simulink model "mdl_4reac_2pump"  (R2020b)
settings: Solver=FixedStepAuto  StartTime=0.0  StopTime=1000  FixedStep=h  MaxStep=1  RelTol=1e-3  AbsTol=1e-6
undefined symbols (not defined in the file or in its folder): p_4reac_2pump
settings Model: PacingRate=0.100000  Creator=nobel  LastModifiedBy=natha

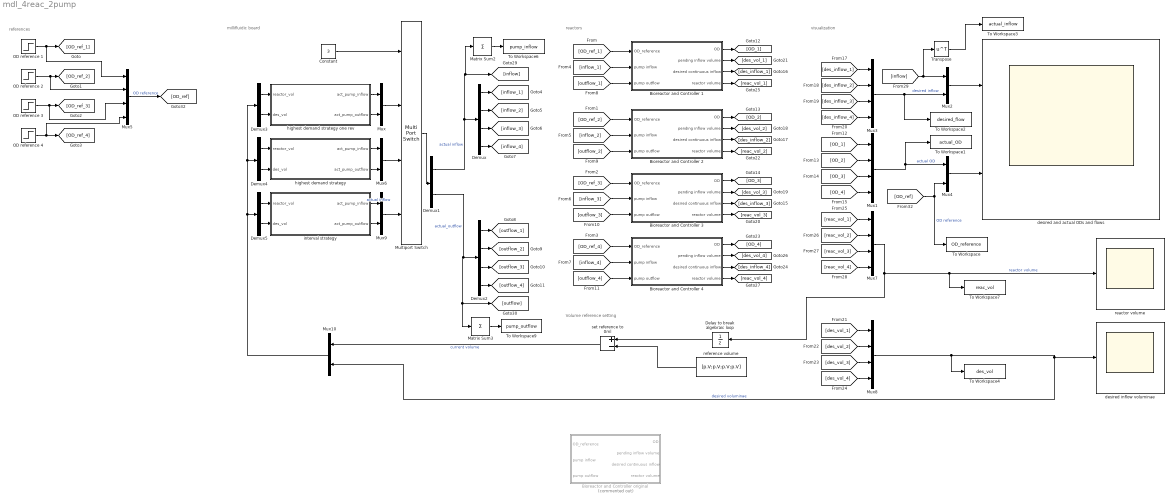
== system mdl_4reac_2pump ==
  note: Volume reference setting
  note: visualization
  note: reactors
  note: millifluidic board
  note: references
  Bioreactor and Controller 1 : Subsystem  mask{p=p_4reac_2pump}
      mask prompts: p "Reactor Parameter Struct"
  Bioreactor and Controller 2 : Subsystem  mask{p=p_4reac_2pump}
      mask prompts: p "Reactor Parameter Struct"
  Bioreactor and Controller 3 : Subsystem  mask{p=p_4reac_2pump}
      mask prompts: p "Reactor Parameter Struct"
  Bioreactor and Controller 4 : Subsystem  mask{p=p_4reac_2pump}
      mask prompts: p "Reactor Parameter Struct"
  Bioreactor and Controller original : Subsystem  Commented=on  mask{p=p_4reac_2pump}
      mask prompts: p "Reactor Parameter Struct"
  Constant : Constant  Value=3
  Delay to break algebraic loop : UnitDelay  InitialCondition=[15; 15; 15; 15]  SampleTime=-1  HasFrameUpgradeWarning=on
  Demux : Demux
  Demux{1,3..5} (4 alike) : Demux  Outputs=2
  Demux2 : Demux
  Matrix Sum2 : Sum  Inputs=+
  Matrix Sum3 : Sum  Inputs=+
  Multiport Switch : MultiPortSwitch
  Mux{,2,4,6,9..10} (6 alike) : Mux  Inputs=2
  Mux{1,3,5,7..8} (5 alike) : Mux
  OD reference 1 : Step  Time=p.r1.step_time  Before=p.r1.init_val  After=p.r1.final_val  SampleTime=0  mask{p=p_4reac_2pump}
      mask prompts: p "Reactor Parameter Struct"
  OD reference 2 : Step  Time=p.r2.step_time  Before=p.r2.init_val  After=p.r2.final_val  SampleTime=0  mask{p=p_4reac_2pump}
      mask prompts: p "Reactor Parameter Struct"
  OD reference 3 : Step  Time=p.r3.step_time  Before=p.r3.init_val  After=p.r3.final_val  SampleTime=0  mask{p=p_4reac_2pump}
      mask prompts: p "Reactor Parameter Struct"
  OD reference 4 : Step  Time=p.r4.step_time  Before=p.r4.init_val  After=p.r4.final_val  SampleTime=0  mask{p=p_4reac_2pump}
      mask prompts: p "Reactor Parameter Struct"
  To Workspace : ToWorkspace  VariableName=OD_reference  SampleTime=-1
  To Workspace1 : ToWorkspace  VariableName=actual_OD  SampleTime=-1
  To Workspace2 : ToWorkspace  VariableName=desired_flow  SampleTime=-1
  To Workspace3 : ToWorkspace  VariableName=actual_inflow  SampleTime=-1
      settings: Save2DSignal=2-D array (concatenate along first dimension)
  To Workspace4 : ToWorkspace  VariableName=des_vol  SampleTime=-1
  To Workspace6 : ToWorkspace  VariableName=pump_inflow  SampleTime=-1
      settings: Save2DSignal=2-D array (concatenate along first dimension)
  To Workspace7 : ToWorkspace  VariableName=reac_vol  SampleTime=-1
  To Workspace9 : ToWorkspace  VariableName=pump_outflow  SampleTime=-1
      settings: Save2DSignal=2-D array (concatenate along first dimension)
  Transpose : Math  Operator=transpose  SaturateOnIntegerOverflow=on
  desired and actual ODs and flows : Scope  NumInputPorts=2
  desired inflow voluminae : Scope
  highest demand strategy : Stateflow chart  TreatAsAtomicUnit=on  mask{p=p_4reac_2pump}
      mask prompts: p "Reactor Parameter Struct"
  highest demand strategy one rev : Stateflow chart  TreatAsAtomicUnit=on  mask{p=p_4reac_2pump}
      mask prompts: p "Reactor Parameter Struct"
  interval strategy : Stateflow chart  TreatAsAtomicUnit=on  mask{p=p_4reac_2pump}
      mask prompts: p "Reactor Parameter Struct"
  reactor volume : Scope
  reference volume : Constant  Value=[p.V;p.V;p.V;p.V]  mask{p=p_4reac_2pump}
      mask prompts: p "Reactor Parameter Struct"
  set reference to 0ml : Sum  Inputs=+-
  wires:
  Bioreactor and Controller 1/2(pending inflow volume) -> [des_vol_1]
  Mux8/1 -> To Workspace4/1, Mux10/2, desired inflow voluminae/1  "desired voluminae"
  Mux1/1 -> To Workspace1/1, Mux4/1  "actual OD"
  Mux2/1 -> desired and actual ODs and flows/1
  Mux3/1 -> To Workspace2/1, Mux2/2  "desired inflow"
  Mux4/1 -> desired and actual ODs and flows/2
  Mux5/1 -> [OD_ref]  "OD reference"
  Demux1/1 -> Matrix Sum2/1, [inflow], Demux/1  "actual inflow"
  Mux7/1 -> Delay to break algebraic loop/1, To Workspace7/1, reactor volume/1  "reactor volume"
  reference volume/1 -> set reference to 0ml/2
  OD reference 1/1 -> Mux5/1, [OD_ref_1]
  OD reference 2/1 -> Mux5/2, [OD_ref_2]
  OD reference 3/1 -> Mux5/3, [OD_ref_3]
  OD reference 4/1 -> Mux5/4, [OD_ref_4]
  [OD_ref_1] -> Bioreactor and Controller 1/1(OD_reference)
  [OD_ref_2] -> Bioreactor and Controller 2/1(OD_reference)
  [OD_ref_3] -> Bioreactor and Controller 3/1(OD_reference)
  [OD_ref_4] -> Bioreactor and Controller 4/1(OD_reference)
  Demux/1 -> [inflow_1]
  Demux/2 -> [inflow_2]
  Demux/3 -> [inflow_3]
  Demux/4 -> [inflow_4]
  [inflow_1] -> Bioreactor and Controller 1/2(pump inflow)
  [inflow_2] -> Bioreactor and Controller 2/2(pump inflow)
  [inflow_3] -> Bioreactor and Controller 3/2(pump inflow)
  [inflow_4] -> Bioreactor and Controller 4/2(pump inflow)
  Demux2/4 -> [outflow_4]
  Demux2/3 -> [outflow_3]
  Demux2/2 -> [outflow_2]
  Demux2/1 -> [outflow_1]
  [outflow_1] -> Bioreactor and Controller 1/3(pump outflow)
  [outflow_2] -> Bioreactor and Controller 2/3(pump outflow)
  [outflow_3] -> Bioreactor and Controller 3/3(pump outflow)
  [outflow_4] -> Bioreactor and Controller 4/3(pump outflow)
  Bioreactor and Controller 1/1(OD) -> [OD_1]
  [OD_1] -> Mux1/1
  [OD_2] -> Mux1/2
  [OD_3] -> Mux1/3
  [OD_4] -> Mux1/4
  [des_inflow_1] -> Mux3/1
  [des_inflow_2] -> Mux3/2
  [des_inflow_3] -> Mux3/3
  [des_inflow_4] -> Mux3/4
  [des_vol_4] -> Mux8/4
  [des_vol_3] -> Mux8/3
  [des_vol_2] -> Mux8/2
  [des_vol_1] -> Mux8/1
  Bioreactor and Controller 1/4(reactor volume) -> [reac_vol_1]
  [reac_vol_1] -> Mux7/1
  [reac_vol_2] -> Mux7/2
  [reac_vol_3] -> Mux7/3
  [reac_vol_4] -> Mux7/4
  Demux1/2 -> Matrix Sum3/1, [outflow], Demux2/1  "actual_outflow"
  [inflow] -> Transpose/1, Mux2/1
  [OD_ref] -> To Workspace/1, Mux4/2  "OD reference"
  Transpose/1 -> To Workspace3/1
  set reference to 0ml/1 -> Mux10/1  "current volume"
  Delay to break algebraic loop/1 -> set reference to 0ml/1
  Bioreactor and Controller 1/3(desired continuous inflow) -> [des_inflow_1]
  Bioreactor and Controller 2/3(desired continuous inflow) -> [des_inflow_2]
  Bioreactor and Controller 2/4(reactor volume) -> [reac_vol_2]
  Bioreactor and Controller 2/1(OD) -> [OD_2]
  Bioreactor and Controller 2/2(pending inflow volume) -> [des_vol_2]
  Bioreactor and Controller 3/2(pending inflow volume) -> [des_vol_3]
  Bioreactor and Controller 3/1(OD) -> [OD_3]
  Bioreactor and Controller 3/4(reactor volume) -> [reac_vol_3]
  Bioreactor and Controller 3/3(desired continuous inflow) -> [des_inflow_3]
  Bioreactor and Controller 4/3(desired continuous inflow) -> [des_inflow_4]
  Bioreactor and Controller 4/4(reactor volume) -> [reac_vol_4]
  Bioreactor and Controller 4/1(OD) -> [OD_4]
  Bioreactor and Controller 4/2(pending inflow volume) -> [des_vol_4]
  Matrix Sum2/1 -> To Workspace6/1
  Matrix Sum3/1 -> To Workspace9/1
  Multiport Switch/1 -> Demux1/1
  highest demand strategy one rev/1(act_pump_inflow) -> Mux/1
  highest demand strategy one rev/2(act_pump_outflow) -> Mux/2
  highest demand strategy/1(act_pump_inflow) -> Mux6/1
  highest demand strategy/2(act_pump_outflow) -> Mux6/2
  interval strategy/1(act_pump_inflow) -> Mux9/1  "actual inflow"
  interval strategy/2(act_pump_outflow) -> Mux9/2
  Mux/1 -> Multiport Switch/2
  Mux6/1 -> Multiport Switch/3
  Mux9/1 -> Multiport Switch/4
  Demux3/1 -> highest demand strategy one rev/1(reactor_vol)
  Demux3/2 -> highest demand strategy one rev/2(des_vol)
  Demux4/1 -> highest demand strategy/1(reactor_vol)
  Demux4/2 -> highest demand strategy/2(des_vol)
  Demux5/1 -> interval strategy/1(reactor_vol)
  Demux5/2 -> interval strategy/2(des_vol)
  Mux10/1 -> Demux5/1, Demux4/1, Demux3/1
  Constant/1 -> Multiport Switch/1

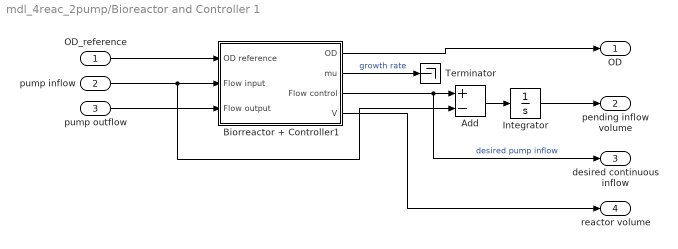
== system mdl_4reac_2pump/Bioreactor and Controller 1 ==
  OD_reference : Inport
  pump inflow : Inport  Port=2
  pump outflow : Inport  Port=3
  Add : Sum  Inputs=+-
  Biorreactor + Controller1 : Subsystem
  Integrator : Integrator
  Terminator : Terminator
  OD : Outport
  pending inflow volume : Outport  Port=2
  desired continuous inflow : Outport  Port=3
  reactor volume : Outport  Port=4
  wires:
  OD_reference/1 -> Biorreactor + Controller1/1(OD reference)
  Biorreactor + Controller1/2(mu) -> Terminator/1  "growth rate"
  Biorreactor + Controller1/1(OD) -> OD/1
  Biorreactor + Controller1/3(Flow control) -> desired continuous inflow/1, Add/1  "desired pump inflow"
  pump inflow/1 -> Add/2, Biorreactor + Controller1/2(Flow input)
  Biorreactor + Controller1/4(V) -> reactor volume/1
  pump outflow/1 -> Biorreactor + Controller1/3(Flow output)
  Add/1 -> Integrator/1
  Integrator/1 -> pending inflow volume/1

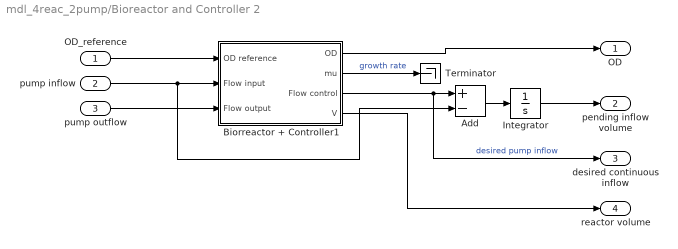
== system mdl_4reac_2pump/Bioreactor and Controller 2 ==
  OD_reference : Inport
  pump inflow : Inport  Port=2
  pump outflow : Inport  Port=3
  Add : Sum  Inputs=+-
  Biorreactor + Controller1 : Subsystem
  Integrator : Integrator
  Terminator : Terminator
  OD : Outport
  pending inflow volume : Outport  Port=2
  desired continuous inflow : Outport  Port=3
  reactor volume : Outport  Port=4
  wires:
  Integrator/1 -> pending inflow volume/1
  Add/1 -> Integrator/1
  pump outflow/1 -> Biorreactor + Controller1/3(Flow output)
  Biorreactor + Controller1/4(V) -> reactor volume/1
  pump inflow/1 -> Biorreactor + Controller1/2(Flow input), Add/2
  Biorreactor + Controller1/3(Flow control) -> Add/1, desired continuous inflow/1  "desired pump inflow"
  Biorreactor + Controller1/1(OD) -> OD/1
  Biorreactor + Controller1/2(mu) -> Terminator/1  "growth rate"
  OD_reference/1 -> Biorreactor + Controller1/1(OD reference)

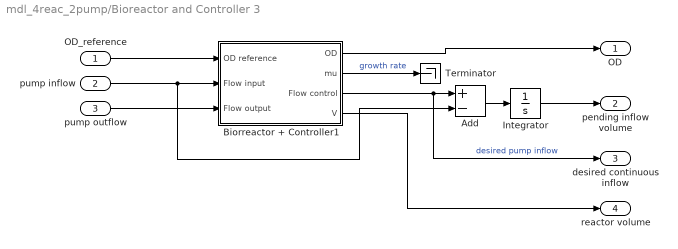
== system mdl_4reac_2pump/Bioreactor and Controller 3 ==
  OD_reference : Inport
  pump inflow : Inport  Port=2
  pump outflow : Inport  Port=3
  Add : Sum  Inputs=+-
  Biorreactor + Controller1 : Subsystem
  Integrator : Integrator
  Terminator : Terminator
  OD : Outport
  pending inflow volume : Outport  Port=2
  desired continuous inflow : Outport  Port=3
  reactor volume : Outport  Port=4
  wires:
  OD_reference/1 -> Biorreactor + Controller1/1(OD reference)
  Biorreactor + Controller1/2(mu) -> Terminator/1  "growth rate"
  Biorreactor + Controller1/1(OD) -> OD/1
  Biorreactor + Controller1/3(Flow control) -> desired continuous inflow/1, Add/1  "desired pump inflow"
  pump inflow/1 -> Add/2, Biorreactor + Controller1/2(Flow input)
  Biorreactor + Controller1/4(V) -> reactor volume/1
  pump outflow/1 -> Biorreactor + Controller1/3(Flow output)
  Add/1 -> Integrator/1
  Integrator/1 -> pending inflow volume/1

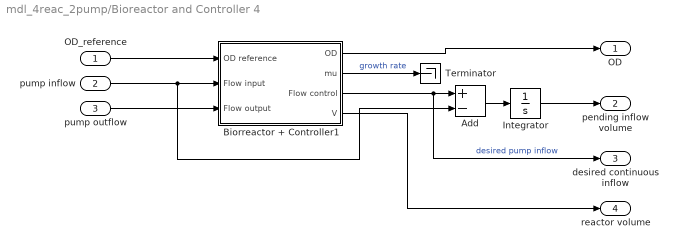
== system mdl_4reac_2pump/Bioreactor and Controller 4 ==
  OD_reference : Inport
  pump inflow : Inport  Port=2
  pump outflow : Inport  Port=3
  Add : Sum  Inputs=+-
  Biorreactor + Controller1 : Subsystem
  Integrator : Integrator
  Terminator : Terminator
  OD : Outport
  pending inflow volume : Outport  Port=2
  desired continuous inflow : Outport  Port=3
  reactor volume : Outport  Port=4
  wires:
  Integrator/1 -> pending inflow volume/1
  Add/1 -> Integrator/1
  pump outflow/1 -> Biorreactor + Controller1/3(Flow output)
  Biorreactor + Controller1/4(V) -> reactor volume/1
  pump inflow/1 -> Biorreactor + Controller1/2(Flow input), Add/2
  Biorreactor + Controller1/3(Flow control) -> Add/1, desired continuous inflow/1  "desired pump inflow"
  Biorreactor + Controller1/1(OD) -> OD/1
  Biorreactor + Controller1/2(mu) -> Terminator/1  "growth rate"
  OD_reference/1 -> Biorreactor + Controller1/1(OD reference)

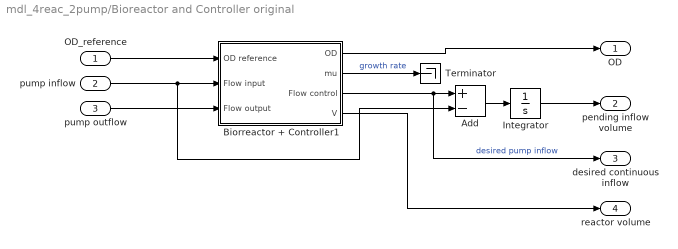
== system mdl_4reac_2pump/Bioreactor and Controller original ==
  OD_reference : Inport
  pump inflow : Inport  Port=2
  pump outflow : Inport  Port=3
  Add : Sum  Inputs=+-
  Biorreactor + Controller1 : Subsystem
  Integrator : Integrator
  Terminator : Terminator
  OD : Outport
  pending inflow volume : Outport  Port=2
  desired continuous inflow : Outport  Port=3
  reactor volume : Outport  Port=4
  wires:
  Integrator/1 -> pending inflow volume/1
  Add/1 -> Integrator/1
  pump outflow/1 -> Biorreactor + Controller1/3(Flow output)
  Biorreactor + Controller1/4(V) -> reactor volume/1
  pump inflow/1 -> Biorreactor + Controller1/2(Flow input), Add/2
  Biorreactor + Controller1/3(Flow control) -> Add/1, desired continuous inflow/1  "desired pump inflow"
  Biorreactor + Controller1/1(OD) -> OD/1
  Biorreactor + Controller1/2(mu) -> Terminator/1  "growth rate"
  OD_reference/1 -> Biorreactor + Controller1/1(OD reference)

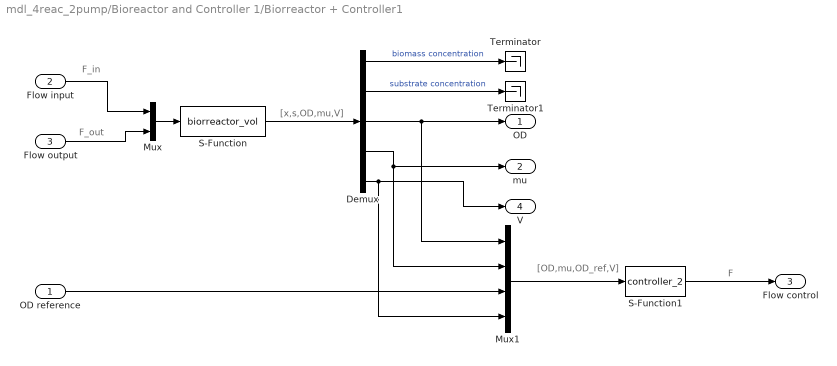
== system mdl_4reac_2pump/Bioreactor and Controller 1/Biorreactor + Controller1 ==
  note: F_out
  note: [OD,mu,OD_ref,V]
  note: F
  note: [x,s,OD,mu,V]
  note: F_in
  OD reference : Inport
  Flow input : Inport  Port=2
  Flow output : Inport  Port=3
  Demux : Demux  Outputs=5
  Mux : Mux  Inputs=2
  Mux1 : Mux
  S-Function : S-Function  FunctionName=biorreactor_vol  Parameters=[0.1 16 15],p  SFunctionDeploymentMode=off  EnableBusSupport=off
  S-Function1 : S-Function  FunctionName=controller_2  Parameters=p  SFunctionDeploymentMode=off  EnableBusSupport=off
  Terminator : Terminator
  Terminator1 : Terminator
  OD : Outport
  mu : Outport  Port=2
  Flow control : Outport  Port=3
  V : Outport  Port=4
  wires:
  Demux/4 -> Mux1/2, mu/1
  Demux/3 -> Mux1/1, OD/1
  OD reference/1 -> Mux1/3
  S-Function/1 -> Demux/1
  Demux/2 -> Terminator1/1  "substrate concentration"
  Mux1/1 -> S-Function1/1
  S-Function1/1 -> Flow control/1
  Demux/1 -> Terminator/1  "biomass concentration"
  Demux/5 -> Mux1/4, V/1
  Mux/1 -> S-Function/1
  Flow input/1 -> Mux/1
  Flow output/1 -> Mux/2

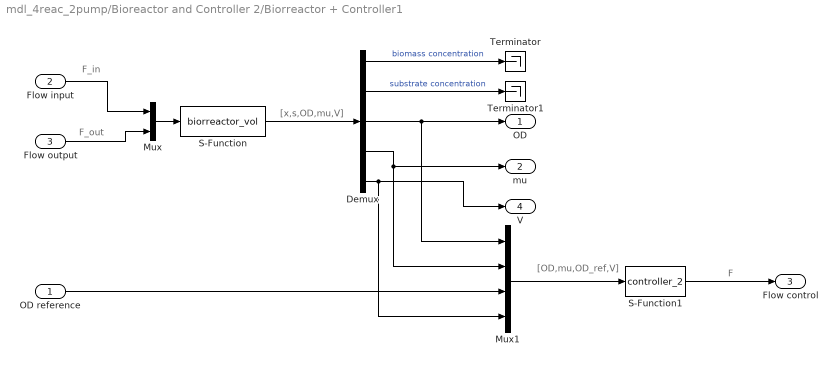
== system mdl_4reac_2pump/Bioreactor and Controller 2/Biorreactor + Controller1 ==
  note: F_in
  note: [x,s,OD,mu,V]
  note: F
  note: [OD,mu,OD_ref,V]
  note: F_out
  OD reference : Inport
  Flow input : Inport  Port=2
  Flow output : Inport  Port=3
  Demux : Demux  Outputs=5
  Mux : Mux  Inputs=2
  Mux1 : Mux
  S-Function : S-Function  FunctionName=biorreactor_vol  Parameters=[0.1 16 15],p  SFunctionDeploymentMode=off  EnableBusSupport=off
  S-Function1 : S-Function  FunctionName=controller_2  Parameters=p  SFunctionDeploymentMode=off  EnableBusSupport=off
  Terminator : Terminator
  Terminator1 : Terminator
  OD : Outport
  mu : Outport  Port=2
  Flow control : Outport  Port=3
  V : Outport  Port=4
  wires:
  Flow output/1 -> Mux/2
  Flow input/1 -> Mux/1
  Mux/1 -> S-Function/1
  Demux/5 -> V/1, Mux1/4
  Demux/1 -> Terminator/1  "biomass concentration"
  S-Function1/1 -> Flow control/1
  Mux1/1 -> S-Function1/1
  Demux/2 -> Terminator1/1  "substrate concentration"
  S-Function/1 -> Demux/1
  OD reference/1 -> Mux1/3
  Demux/3 -> OD/1, Mux1/1
  Demux/4 -> mu/1, Mux1/2

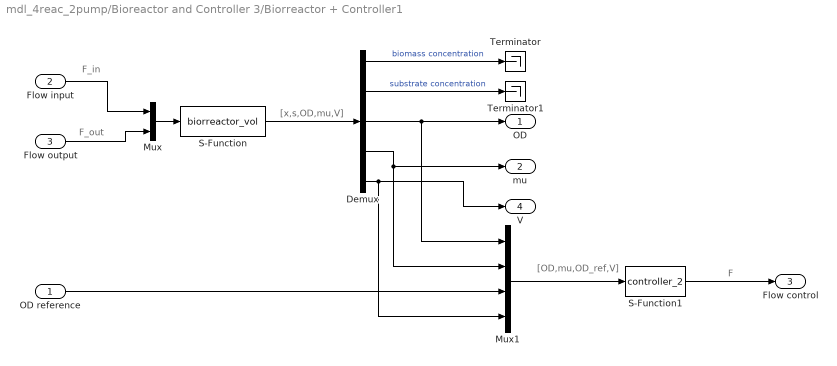
== system mdl_4reac_2pump/Bioreactor and Controller 3/Biorreactor + Controller1 ==
  note: F_out
  note: [OD,mu,OD_ref,V]
  note: F
  note: [x,s,OD,mu,V]
  note: F_in
  OD reference : Inport
  Flow input : Inport  Port=2
  Flow output : Inport  Port=3
  Demux : Demux  Outputs=5
  Mux : Mux  Inputs=2
  Mux1 : Mux
  S-Function : S-Function  FunctionName=biorreactor_vol  Parameters=[0.1 16 15],p  SFunctionDeploymentMode=off  EnableBusSupport=off
  S-Function1 : S-Function  FunctionName=controller_2  Parameters=p  SFunctionDeploymentMode=off  EnableBusSupport=off
  Terminator : Terminator
  Terminator1 : Terminator
  OD : Outport
  mu : Outport  Port=2
  Flow control : Outport  Port=3
  V : Outport  Port=4
  wires:
  Demux/4 -> Mux1/2, mu/1
  Demux/3 -> Mux1/1, OD/1
  OD reference/1 -> Mux1/3
  S-Function/1 -> Demux/1
  Demux/2 -> Terminator1/1  "substrate concentration"
  Mux1/1 -> S-Function1/1
  S-Function1/1 -> Flow control/1
  Demux/1 -> Terminator/1  "biomass concentration"
  Demux/5 -> Mux1/4, V/1
  Mux/1 -> S-Function/1
  Flow input/1 -> Mux/1
  Flow output/1 -> Mux/2

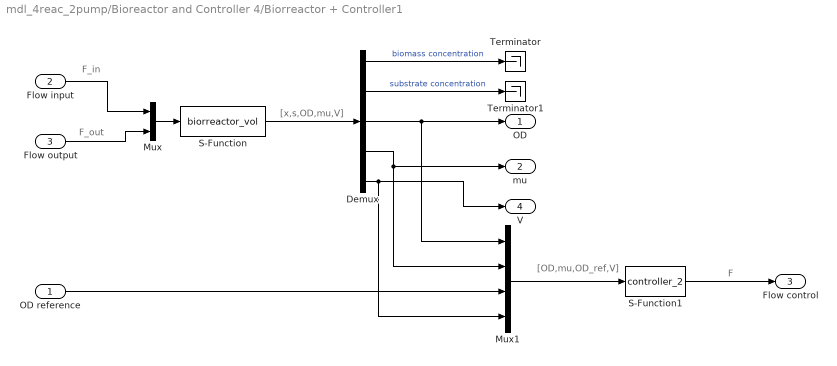
== system mdl_4reac_2pump/Bioreactor and Controller 4/Biorreactor + Controller1 ==
  note: F_in
  note: [x,s,OD,mu,V]
  note: F
  note: [OD,mu,OD_ref,V]
  note: F_out
  OD reference : Inport
  Flow input : Inport  Port=2
  Flow output : Inport  Port=3
  Demux : Demux  Outputs=5
  Mux : Mux  Inputs=2
  Mux1 : Mux
  S-Function : S-Function  FunctionName=biorreactor_vol  Parameters=[0.1 16 15],p  SFunctionDeploymentMode=off  EnableBusSupport=off
  S-Function1 : S-Function  FunctionName=controller_2  Parameters=p  SFunctionDeploymentMode=off  EnableBusSupport=off
  Terminator : Terminator
  Terminator1 : Terminator
  OD : Outport
  mu : Outport  Port=2
  Flow control : Outport  Port=3
  V : Outport  Port=4
  wires:
  Flow output/1 -> Mux/2
  Flow input/1 -> Mux/1
  Mux/1 -> S-Function/1
  Demux/5 -> V/1, Mux1/4
  Demux/1 -> Terminator/1  "biomass concentration"
  S-Function1/1 -> Flow control/1
  Mux1/1 -> S-Function1/1
  Demux/2 -> Terminator1/1  "substrate concentration"
  S-Function/1 -> Demux/1
  OD reference/1 -> Mux1/3
  Demux/3 -> OD/1, Mux1/1
  Demux/4 -> mu/1, Mux1/2

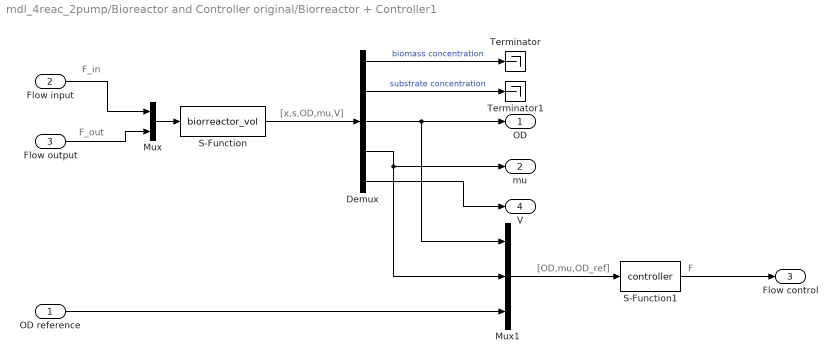
== system mdl_4reac_2pump/Bioreactor and Controller original/Biorreactor + Controller1 ==
  note: F_in
  note: [x,s,OD,mu,V]
  note: F
  note: [OD,mu,OD_ref]
  note: F_out
  OD reference : Inport
  Flow input : Inport  Port=2
  Flow output : Inport  Port=3
  Demux : Demux  Outputs=5
  Mux : Mux  Inputs=2
  Mux1 : Mux  Inputs=3
  S-Function : S-Function  FunctionName=biorreactor_vol  Parameters=[0.1 16 15],p  SFunctionDeploymentMode=off  EnableBusSupport=off
  S-Function1 : S-Function  FunctionName=controller  Parameters=p  SFunctionDeploymentMode=off  EnableBusSupport=off
  Terminator : Terminator
  Terminator1 : Terminator
  OD : Outport
  mu : Outport  Port=2
  Flow control : Outport  Port=3
  V : Outport  Port=4
  wires:
  Flow output/1 -> Mux/2
  Flow input/1 -> Mux/1
  Mux/1 -> S-Function/1
  Demux/5 -> V/1
  Demux/1 -> Terminator/1  "biomass concentration"
  S-Function1/1 -> Flow control/1
  Mux1/1 -> S-Function1/1
  Demux/2 -> Terminator1/1  "substrate concentration"
  S-Function/1 -> Demux/1
  OD reference/1 -> Mux1/3
  Demux/3 -> OD/1, Mux1/1
  Demux/4 -> mu/1, Mux1/2

== stateflow chart mdl_4reac_2pump/highest demand strategy one rev ==
  state procedures [parallel]
    settings: executionOrder=1
    state normal
    state sampling
      entry: sampling_req=true;
    (default) -> normal
    normal -> sampling : after(15, sec)
    sampling -> normal : sampling_done
  state feeding [parallel]
    settings: executionOrder=2
    state inflow
      state inflow_act
        entry: act_pump_inflow(reac_ind_inflow)=...
        p.max_pump_flow;
      state inflow_inact
        entry: act_pump_inflow=zeros(4,1);
        [vol_pump_in, reac_ind_inflow] = max(des_vol);
        during: [vol_pump_in, reac_ind_inflow] = max(des_vol);
      inflow_act -> inflow_inact : after(p.pump_res/p.max_pump_flow,sec)
      inflow_inact -> inflow_act : [vol_pump_in>=p.pump_res]
    (default) -> inflow_inact
  state wasting_sampling [parallel]
    settings: executionOrder=3
    state outflow_waste
      state outflow_act
        entry: act_pump_outflow(reac_ind_outflow)=...
        p.max_pump_flow;
      state outflow_inact
        entry: act_pump_outflow=zeros(4,1);
        [vol_pump_out, reac_ind_outflow] = max(reactor_vol);
        during: [vol_pump_out, reac_ind_outflow] = ...
        max(reactor_vol);
      wasting_sampling.outflow_waste.outflow_act -> wasting_sampling.outflow_waste.outflow_inact [order 1] : after(vol_pump_out/p.max_pump_flow,sec)
      wasting_sampling.outflow_waste.outflow_act -> wasting_sampling.outflow_waste.outflow_inact [order 2] : [vol_pump_out<=0]
      wasting_sampling.outflow_waste.outflow_inact -> wasting_sampling.outflow_waste.outflow_act [order 2] : [vol_pump_out>=p.pump_res]
    state cleaning_procedure
    state outflow_sampling
      state outflow_act
        entry: vol_pump_out=p.pump_res;
        act_pump_outflow(reac_ind_outflow)=p.max_pump_flow;
      state outflow_inact
        entry: act_pump_outflow=zeros(4,1);
      wasting_sampling.outflow_sampling.outflow_act -> wasting_sampling.outflow_sampling.outflow_inact : after(vol_pump_out/p.max_pump_flow,sec)
      wasting_sampling.outflow_sampling.outflow_inact -> wasting_sampling.outflow_sampling.outflow_act [order 2] : {reac_ind_outflow=reac_ind_outflow+1;}
    (default) -> wasting_sampling.outflow_waste.outflow_inact
    wasting_sampling.outflow_waste.outflow_inact -> cleaning_procedure [order 1] : [in(procedures.sampling)]
    wasting_sampling.outflow_sampling.outflow_inact -> wasting_sampling.outflow_waste.outflow_inact [order 1] : [reac_ind_outflow==4]{send(sampling_done,procedures)}
    cleaning_procedure -> (junction 263) : after(p.clean_time,sec)
    (junction 263) -> wasting_sampling.outflow_sampling.outflow_act : {reac_ind_outflow=1;}
  data: act_pump_inflow output =[0;0;0;0]; reactor_vol input; des_vol input size=4; vol_pump_in local; act_pump_outflow output =[0;0;0;0]; vol_pump_out local; reac_ind_inflow local =1; sampling_req local; p parameter; reac_ind_outflow local =1
  events: sampling_done local FUNCTION_CALL_EVENT

== stateflow chart mdl_4reac_2pump/highest demand strategy ==
  state procedures [parallel]
    settings: executionOrder=1
    state normal
    state sampling
      entry: sampling_req=true;
    (default) -> normal
    normal -> sampling : after(15, sec)
    sampling -> normal : sampling_done
  state feeding [parallel]
    settings: executionOrder=2
    state inflow
      state inflow_act
        entry: act_pump_inflow(reac_ind_inflow)=...
        p.max_pump_flow;
        vol_pump_in = floor(vol_pump_out/p.pump_res)...
        *p.pump_res;
      state inflow_inact
        entry: act_pump_inflow=zeros(4,1);
        [vol_pump_in, reac_ind_inflow] = max(des_vol);
        during: [vol_pump_in, reac_ind_inflow] = max(des_vol);
      inflow_act -> inflow_inact [order 1] : after(vol_pump_in/p.max_pump_flow,sec)
      inflow_act -> inflow_inact [order 2] : [vol_pump_in<=0]
      inflow_inact -> inflow_act : [vol_pump_in>=p.pump_res]
    (default) -> inflow_inact
  state wasting_sampling [parallel]
    settings: executionOrder=3
    state outflow_waste
      state outflow_act
        entry: act_pump_outflow(reac_ind_outflow)=...
        p.max_pump_flow;
        % vol_pump_out = floor(vol_pump_out/p.pump_res)...
        % *p.pump_res;
      state outflow_inact
        entry: act_pump_outflow=zeros(4,1);
        [vol_pump_out, reac_ind_outflow] = max(reactor_vol);
        during: [vol_pump_out, reac_ind_outflow] = ...
        max(reactor_vol);
      wasting_sampling.outflow_waste.outflow_act -> wasting_sampling.outflow_waste.outflow_inact [order 1] : after(vol_pump_out/p.max_pump_flow,sec)
      wasting_sampling.outflow_waste.outflow_act -> wasting_sampling.outflow_waste.outflow_inact [order 2] : [vol_pump_out<=0]
      wasting_sampling.outflow_waste.outflow_inact -> wasting_sampling.outflow_waste.outflow_act [order 2] : [vol_pump_out>=p.pump_res]
    state cleaning_procedure
    state outflow_sampling
      state outflow_act
        entry: vol_pump_out=p.pump_res;
        act_pump_outflow(reac_ind_outflow)=p.max_pump_flow;
      state outflow_inact
        entry: act_pump_outflow=zeros(4,1);
      wasting_sampling.outflow_sampling.outflow_act -> wasting_sampling.outflow_sampling.outflow_inact : after(vol_pump_out/p.max_pump_flow,sec)
      wasting_sampling.outflow_sampling.outflow_inact -> wasting_sampling.outflow_sampling.outflow_act [order 2] : {reac_ind_outflow=reac_ind_outflow+1;}
    (default) -> wasting_sampling.outflow_waste.outflow_inact
    wasting_sampling.outflow_waste.outflow_inact -> cleaning_procedure [order 1] : [in(procedures.sampling)]
    wasting_sampling.outflow_sampling.outflow_inact -> wasting_sampling.outflow_waste.outflow_inact [order 1] : [reac_ind_outflow==4]{send(sampling_done,procedures)}
    cleaning_procedure -> (junction 263) : after(p.clean_time,sec)
    (junction 263) -> wasting_sampling.outflow_sampling.outflow_act : {reac_ind_outflow=1;}
  data: act_pump_inflow output =[0;0;0;0]; reactor_vol input; des_vol input size=4; vol_pump_in local; act_pump_outflow output =[0;0;0;0]; vol_pump_out local; reac_ind_inflow local =1; sampling_req local; p parameter; reac_ind_outflow local =1
  events: sampling_done local FUNCTION_CALL_EVENT

== stateflow chart mdl_4reac_2pump/interval strategy ==
  state counter_inflow [parallel]
    settings: executionOrder=1
    state init_counter
      entry: reac_ind_inflow = 1;
    state increase_counter
      entry: reac_ind_inflow = reac_ind_inflow+1;
    state cycle_over
    (default) -> counter_inflow.init_counter : % loop_counter
    (junction 211) -> counter_inflow.cycle_over [order 2]
    (junction 211) -> counter_inflow.increase_counter [order 1] : [reac_ind_inflow<p.num_reac]
    counter_inflow.increase_counter -> (junction 211) : after(p.interval/p.num_reac,sec)
    counter_inflow.init_counter -> counter_inflow.increase_counter : after(p.interval/p.num_reac,sec)
    counter_inflow.cycle_over -> counter_inflow.init_counter
  state procedures [parallel]
    settings: executionOrder=3
    state normal
    state sampling
      entry: sampling_req=true;
    (default) -> normal
    normal -> sampling : after(15, sec)
    sampling -> normal : sampling_done
  state counter_outflow [parallel]
    settings: executionOrder=4
    state init_counter
      entry: reac_ind_outflow = 1;
    state increase_counter
      entry: reac_ind_outflow = reac_ind_outflow+1;
    state cycle_over
    (default) -> counter_outflow.init_counter : % loop_counter
    (junction 274) -> counter_outflow.cycle_over [order 2]
    (junction 274) -> counter_outflow.increase_counter [order 1] : [reac_ind_outflow<p.num_reac]
    counter_outflow.increase_counter -> (junction 274) : after(p.interval/p.num_reac,sec)
    counter_outflow.init_counter -> counter_outflow.increase_counter : after(p.interval/p.num_reac,sec)
    counter_outflow.cycle_over -> counter_outflow.init_counter : next_cycle
  state feeding [parallel]
    settings: executionOrder=5
    state inflow
      state inflow_act
        entry: vol_pump_in=floor(des_vol(reac_ind_inflow)/...
        p.pump_res)*p.pump_res;
        act_pump_inflow(reac_ind_inflow)=p.max_pump_flow;
      state inflow_inact
        entry: act_pump_inflow=zeros(4,1);
      inflow_act -> inflow_inact [order 3] : [vol_pump_in<=0]
      inflow_act -> inflow_inact [order 1] : after(vol_pump_in/p.max_pump_flow,sec)
      inflow_inact -> inflow_act [order 1] : enter(counter_inflow.increase_counter)
      inflow_inact -> inflow_act [order 2] : enter(counter_inflow.init_counter)
      inflow_act -> inflow_inact [order 2] : after(p.interval/p.num_reac-1e-3,sec)
    (default) -> inflow_act
  state wasting_sampling [parallel]
    settings: executionOrder=2
    state outflow_waste
      state outflow_act
        entry:vol_pump_out = reactor_vol(reac_ind_outflow);
        %vol_pump_out=...
        %  floor(reactor_vol(reac_ind_outflow)/...
        %  p.pump_res)*p.pump_res;
        act_pump_outflow(reac_ind_outflow)=p.max_pump_flow;
      state outflow_inact
        entry: act_pump_outflow=zeros(4,1);
      wasting_sampling.outflow_waste.outflow_inact -> wasting_sampling.outflow_waste.outflow_act [order 1] : [enter(counter_outflow.cycle_over) && in(procedures.normal)]{send(next_cycle,counter_outflow)}
      wasting_sampling.outflow_waste.outflow_act -> wasting_sampling.outflow_waste.outflow_inact [order 1] : [vol_pump_out<=0]
      wasting_sampling.outflow_waste.outflow_act -> wasting_sampling.outflow_waste.outflow_inact [order 2] : after(vol_pump_out/p.max_pump_flow,sec)
      wasting_sampling.outflow_waste.outflow_inact -> wasting_sampling.outflow_waste.outflow_act [order 2] : enter(counter_outflow.increase_counter)
      wasting_sampling.outflow_waste.outflow_act -> wasting_sampling.outflow_waste.outflow_inact [order 3] : after(p.interval/p.num_reac-1e-3,sec)
    state cleaning_procedure
    state outflow_sampling
      state outflow_act
        entry: vol_pump_out=p.pump_res;
        act_pump_outflow(reac_ind_outflow)=...
        p.max_pump_flow;
      state outflow_inact
        entry: act_pump_outflow=zeros(4,1);
      wasting_sampling.outflow_sampling.outflow_act -> wasting_sampling.outflow_sampling.outflow_inact : after(vol_pump_out/p.max_pump_flow,sec)
      wasting_sampling.outflow_sampling.outflow_inact -> wasting_sampling.outflow_sampling.outflow_act [order 1] : enter(counter_outflow.increase_counter)
    (default) -> wasting_sampling.outflow_waste.outflow_act
    wasting_sampling.outflow_waste.outflow_inact -> cleaning_procedure [order 3] : [enter(counter_outflow.cycle_over) && in(procedures.sampling)]
    wasting_sampling.outflow_sampling.outflow_inact -> wasting_sampling.outflow_waste.outflow_act [order 2] : [enter(counter_outflow.cycle_over)]{send(sampling_done, procedures);send(next_cycle, counter_outflow)}
    cleaning_procedure -> (junction 263) : after(p.clean_time,sec)
    (junction 263) -> wasting_sampling.outflow_sampling.outflow_act : {send(next_cycle,counter_outflow)}
  data: act_pump_inflow output =[0;0;0;0]; reactor_vol input; des_vol input size=4; vol_pump_in local; act_pump_outflow output =[0;0;0;0]; vol_pump_out local; reac_ind_inflow local =1; sampling_req local; p parameter; reac_ind_outflow local =1
  events: sampling_done local FUNCTION_CALL_EVENT; next_cycle local FUNCTION_CALL_EVENT
